simulink model "heat_exchanger_disassembled"  (R2017b)
settings: Solver=VariableStepAuto  StartTime=0.0  StopTime=20  RelTol=1e-3
undefined symbols (not defined in the file): Area, cp_H2O, cp_wort, HE_delay, m_H2O, m_wort, Reference, T_H2O_in, T_wort_in, U
settings Model: Creator=Alexander  LastModifiedBy=Alexander

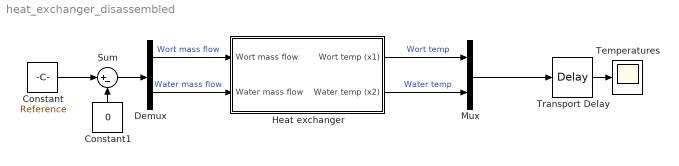
== system heat_exchanger_disassembled ==
  Constant : Constant  Value=Reference
  Constant1 : Constant  Value=0
  Demux : Demux  Outputs=2
  Heat exchanger : Subsystem
  Mux : Mux  Inputs=2
  Sum : Sum  Inputs=|+-
  Temperatures : Scope
  Transport Delay : TransportDelay  DelayTime=HE_delay
  wires:
  Transport Delay/1 -> Temperatures/1
  Heat exchanger/2(Water temp (x2)) -> Mux/2  "Water temp"
  Heat exchanger/1(Wort temp (x1)) -> Mux/1  "Wort temp"
  Mux/1 -> Transport Delay/1
  Constant/1 -> Sum/1
  Demux/2 -> Heat exchanger/2(Water mass flow)  "Water mass flow"
  Demux/1 -> Heat exchanger/1(Wort mass flow)  "Wort mass flow"
  Sum/1 -> Demux/1
  Constant1/1 -> Sum/2

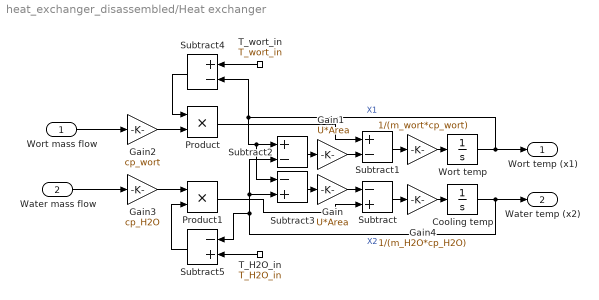
== system heat_exchanger_disassembled/Heat exchanger ==
  Wort mass flow : Inport
  Water mass flow : Inport  Port=2
  " " : Gain  Gain=1/(m_wort*cp_wort)
  Cooling temp : Integrator  InitialCondition=T_H2O_in
  Gain : Gain  Gain=U*Area
  Gain1 : Gain  Gain=U*Area
  Gain2 : Gain  Gain=cp_wort
  Gain3 : Gain  Gain=cp_H2O
  Gain4 : Gain  Gain=1/(m_H2O*cp_H2O)
  Product : Product
  Product1 : Product
  Subtract : Sum  Inputs=-+
  Subtract1 : Sum  Inputs=+-
  Subtract2 : Sum  Inputs=+-
  Subtract3 : Sum  Inputs=-+
  Subtract4 : Sum  Inputs=+-
  Subtract5 : Sum  Inputs=-+
  T_H2O_in : Constant  Value=T_H2O_in
  T_wort_in : Constant  Value=T_wort_in
  Wort temp : Integrator  InitialCondition=T_wort_in
  Wort temp (x1) : Outport
  Water temp (x2) : Outport  Port=2
  wires:
  Cooling temp/1 -> Water temp (x2)/1, Subtract5/1, Subtract3/2, Subtract2/2  "X2"
  " "/1 -> Wort temp/1
  Wort temp/1 -> Subtract4/2, Subtract3/1, Subtract2/1, Wort temp (x1)/1  "X1"
  Gain1/1 -> Subtract1/2
  Subtract1/1 -> " "/1
  Gain4/1 -> Cooling temp/1
  Gain/1 -> Subtract/1
  Subtract2/1 -> Gain1/1
  Subtract3/1 -> Gain/1
  Subtract/1 -> Gain4/1
  Wort mass flow/1 -> Gain2/1
  T_wort_in/1 -> Subtract4/1
  Subtract5/1 -> Product1/2
  Product/1 -> Subtract1/1
  T_H2O_in/1 -> Subtract5/2
  Subtract4/1 -> Product/1
  Product1/1 -> Subtract/2
  Water mass flow/1 -> Gain3/1
  Gain3/1 -> Product1/1
  Gain2/1 -> Product/2
